simulink model "msePardoSplitOfFour"  (R2024b)
settings: Solver=VariableStepAuto  StartTime=0.0  StopTime=10.0  RelTol=1e-3
settings Model: Creator=DarianMuresan  LastModifiedBy=ferbe
settings RTWCC: GPUComputeCapability=3.5

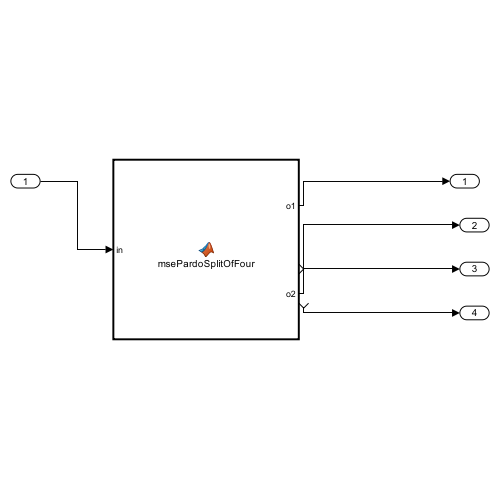
[thumbnail: Simulink's stored preview of the top-level diagram]
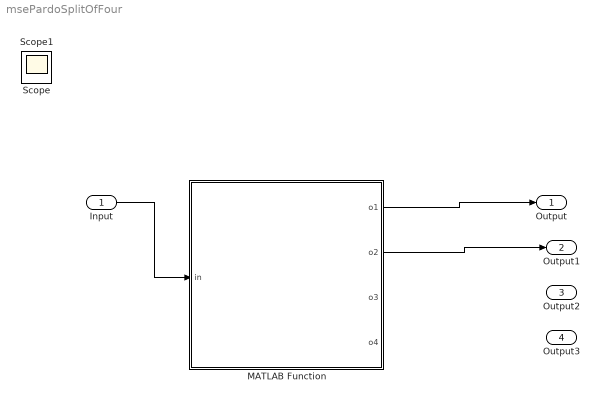
== system msePardoSplitOfFour ==
  Input : Inport
  MATLAB Function : MATLAB Function  TreatAsAtomicUnit=on
  Output : Outport
  Output1 : Outport  Port=2
  Output2 : Outport  Port=3
  Output3 : Outport  Port=4
  Scope : Scope
  Scope1 : Scope
  wires:
  MATLAB Function/1(o1) -> Output/1
  MATLAB Function/2(o2) -> Output1/1
  ? -> Output2/1
  ? -> Output3/1
  Input/1 -> MATLAB Function/1(in)

== matlab function msePardoSplitOfFour/MATLAB Function ==
  data: in input; o1 output; o2 output; o3 output; o4 output
function [o1,o2,o3,o4] = msePardoSplitOfFour(in)

% Method to demux input into one of 4 possible outputs based on
% the assumption that processes run in parallel and they must all complete.
%
% A non-valid output is negative
%
% Written by: Darian Muresan
% Last Modified: 10/10/2024

if in<0
    o1 = -1;
    o2 = -1;
    o3 = -1;
    o4 = -1;
else
    o1 = in;
    o2 = in;
    o3 = in;
    o4 = in;    
end
